simulink model "EX3_zadanie1_zadanie2"  (R2023b)
settings: Solver=FixedStepDiscrete  StartTime=0.0  StopTime=0.0  RelTol=1e-3
libraries: CPOiS_SourcesSinks x12, CPOiS_LinearTransforms x6, CPOiS_DataManipulation_DataTypeConversion x3
settings Model: Creator=alyskawa  LastModifiedBy=alyskawa

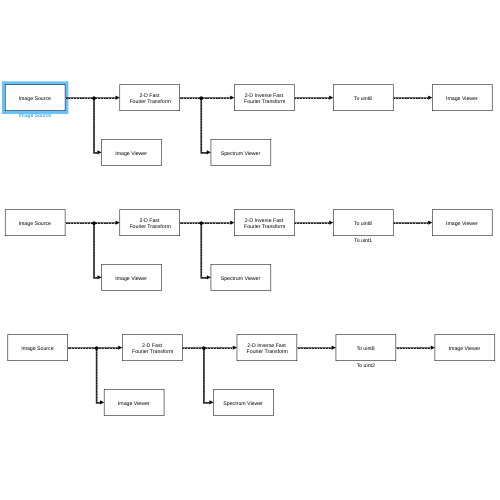
[thumbnail: Simulink's stored preview of the top-level diagram]
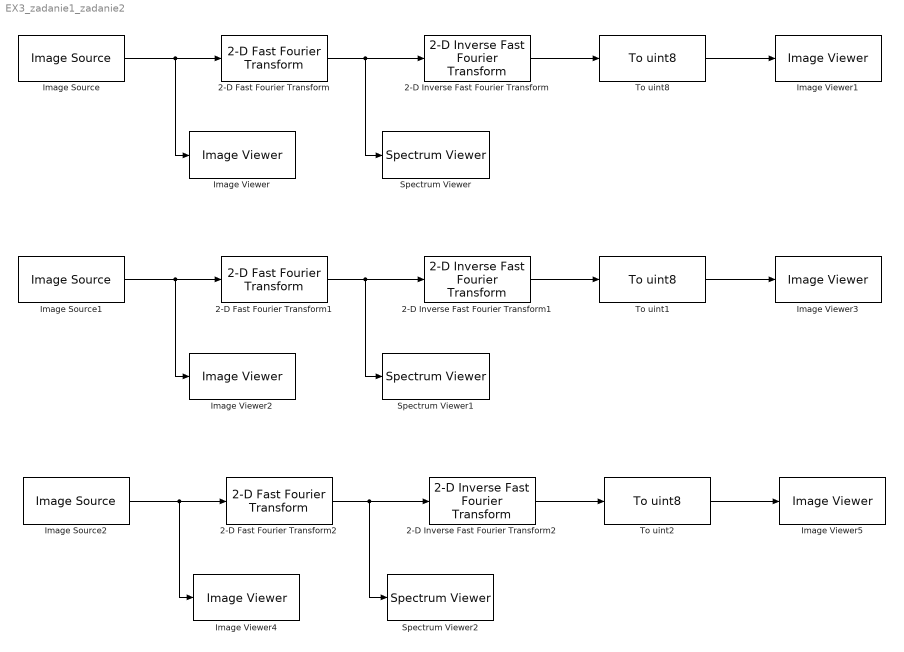
== system EX3_zadanie1_zadanie2 ==
  2-D Fast Fourier Transform : CPOiS_LinearTransforms/2-D Fast Fourier Transform
      settings: SourceProductName=CPOiS - Digital image and signal processing
  2-D Fast Fourier Transform1 : CPOiS_LinearTransforms/2-D Fast Fourier Transform
      settings: SourceProductName=CPOiS - Digital image and signal processing
  2-D Fast Fourier Transform2 : CPOiS_LinearTransforms/2-D Fast Fourier Transform
      settings: SourceProductName=CPOiS - Digital image and signal processing
  2-D Inverse Fast Fourier Transform : CPOiS_LinearTransforms/2-D Inverse Fast  Fourier Transform
      settings: SourceProductName=CPOiS - Digital image and signal processing
  2-D Inverse Fast Fourier Transform1 : CPOiS_LinearTransforms/2-D Inverse Fast  Fourier Transform
      settings: SourceProductName=CPOiS - Digital image and signal processing
  2-D Inverse Fast Fourier Transform2 : CPOiS_LinearTransforms/2-D Inverse Fast  Fourier Transform
      settings: SourceProductName=CPOiS - Digital image and signal processing
  Image Source : CPOiS_SourcesSinks/Image Source  FileSelection=marine.png
      settings: SourceProductName=CPOiS - Digital image and signal processing
  Image Source1 : CPOiS_SourcesSinks/Image Source  FileSelection=marine.png
      settings: SourceProductName=CPOiS - Digital image and signal processing
  Image Source2 : CPOiS_SourcesSinks/Image Source  FileSelection=gull.png
      settings: SourceProductName=CPOiS - Digital image and signal processing
  Image Viewer{,1..5} (6 alike) : CPOiS_SourcesSinks/Image Viewer
      settings: SourceProductName=CPOiS - Digital image and signal processing
  Spectrum Viewer : CPOiS_SourcesSinks/Spectrum Viewer
      settings: SourceProductName=CPOiS - Digital image and signal processing
  Spectrum Viewer1 : CPOiS_SourcesSinks/Spectrum Viewer
      settings: SourceProductName=CPOiS - Digital image and signal processing
  Spectrum Viewer2 : CPOiS_SourcesSinks/Spectrum Viewer
      settings: SourceProductName=CPOiS - Digital image and signal processing
  To uint1 : CPOiS_DataManipulation_DataTypeConversion/To uint8
      settings: SourceProductName=CPOiS - Digital image and signal processing
  To uint2 : CPOiS_DataManipulation_DataTypeConversion/To uint8
      settings: SourceProductName=CPOiS - Digital image and signal processing
  To uint8 : CPOiS_DataManipulation_DataTypeConversion/To uint8
      settings: SourceProductName=CPOiS - Digital image and signal processing
  wires:
  Image Source/1 -> Image Viewer/1, 2-D Fast Fourier Transform/1
  2-D Fast Fourier Transform/1 -> Spectrum Viewer/1, 2-D Inverse Fast Fourier Transform/1
  2-D Inverse Fast Fourier Transform/1 -> To uint8/1
  To uint8/1 -> Image Viewer1/1
  2-D Fast Fourier Transform1/1 -> Spectrum Viewer1/1, 2-D Inverse Fast Fourier Transform1/1
  2-D Inverse Fast Fourier Transform1/1 -> To uint1/1
  To uint1/1 -> Image Viewer3/1
  Image Source1/1 -> Image Viewer2/1, 2-D Fast Fourier Transform1/1
  2-D Fast Fourier Transform2/1 -> Spectrum Viewer2/1, 2-D Inverse Fast Fourier Transform2/1
  2-D Inverse Fast Fourier Transform2/1 -> To uint2/1
  To uint2/1 -> Image Viewer5/1
  Image Source2/1 -> Image Viewer4/1, 2-D Fast Fourier Transform2/1
